simulink model "sampleModel1917"  (R2023a)
settings: Solver=VariableStepAuto  StartTime=0.0  StopTime=10.0  RelTol=1e-3
libraries: hdlsllib x8, simulink x8
settings Model: Creator=user1  LastModifiedBy=user1

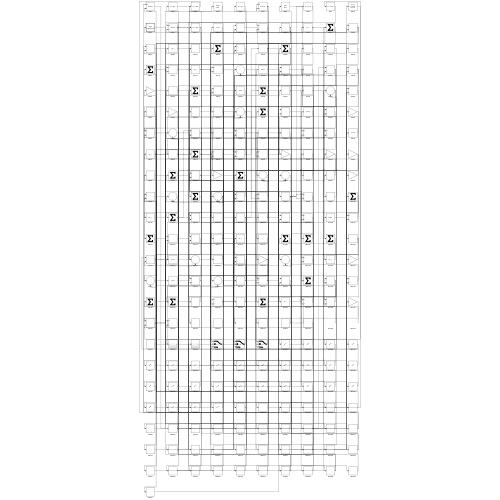
[thumbnail: Simulink's stored preview of the top-level diagram]
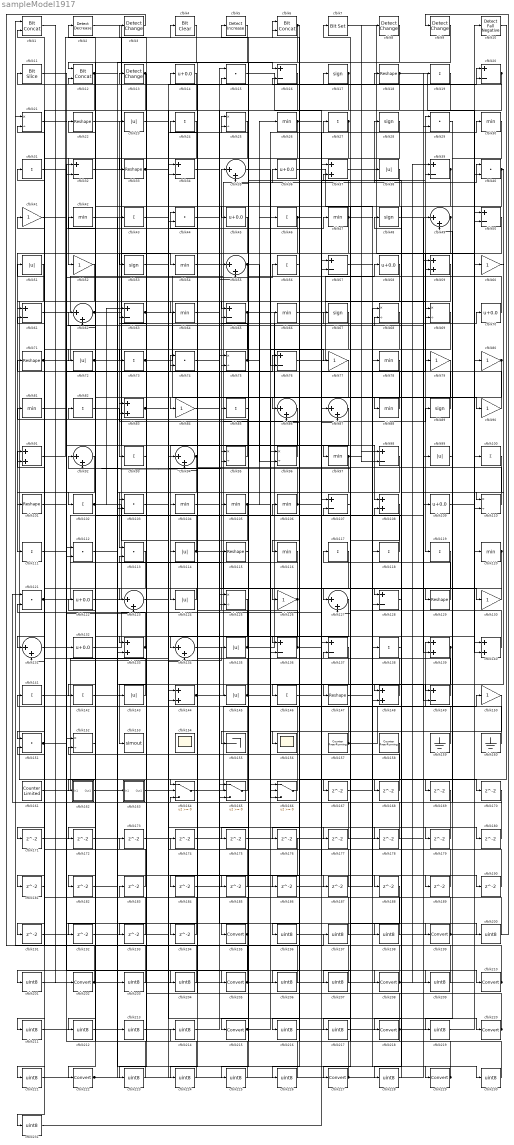
== system sampleModel1917 ==
  cfblk1 : hdlsllib/Logic and Bit Operations/Bit Concat  numInputs=2
  cfblk10 : hdlsllib/Logic and Bit Operations/Detect Fall Negative  vinit=0  OutDataTypeStr=boolean
  cfblk{19,24,27,31,43,46,56,73,82,85,93,100,102,111,117..119,138,141..142,146} (21 alike) : Sum  Inputs=+
  cfblk{18,22,33,71,101,115,129,147} (8 alike) : Reshape
  cfblk{15,29,40,44,74,103,112..113,121,151} (10 alike) : DotProduct  OutDataTypeStr=Inherit: Inherit via internal rule
  cfblk{26,30,42,47,54,64,66,78,81,88,97,104..106,116,120} (16 alike) : MinMax
  cfblk{16,20,32,34,39,50,57,61,63,65,76,98,107,128,136..137,149} (17 alike) : Sum  Inputs=+-
  cfblk{37,59,83,91,108,133,139..140,144,148} (10 alike) : Sum
  cfblk{14,36,45,58,70,109,122,132} (8 alike) : Bias  Bias=0.0  SaturateOnIntegerOverflow=off
  cfblk11 : hdlsllib/Logic and Bit Operations/Bit Slice  lidx=7  ridx=0
  cfblk{21,25,68..69,75,95..96,110,125,152} (10 alike) : Product  Inputs=*/  RndMeth=Zero  SaturateOnIntegerOverflow=on
  cfblk{23,38,51,72,99,114,124,135,143,145} (10 alike) : Abs  SaturateOnIntegerOverflow=off
  cfblk12 : hdlsllib/Logic and Bit Operations/Bit Concat  numInputs=2
  cfblk{35,49,55,62,86..87,92,94,123,127,131,134} (12 alike) : Sum  Inputs=|++
  cfblk{41,52,60,77,79..80,84,90,126,130,150} (11 alike) : Gain
  cfblk{3,8..9,13} (4 alike) : simulink/Logic and Bit Operations/Detect Change  vinit=0  OutDataTypeStr=boolean
      settings: LibrarySourceBlock=|
      | hdlsllib/Logic and Bit
      | Operations/Detect
      | Change
  cfblk153 : ToWorkspace  VariableName=simout  SaveFormat=Timeseries  SampleTime=-1
  cfblk154 : Scope
      settings: Floating=on
  cfblk155 : Terminator
  cfblk156 : Scope
  cfblk157 : hdlsllib/Sources/Counter Free-Running  NumBits=16  tsamp=-1
  cfblk158 : hdlsllib/Sources/Counter Free-Running  NumBits=16  tsamp=-1
  cfblk159 : Ground
  cfblk160 : Ground
  cfblk161 : hdlsllib/Sources/Counter Limited  uplimit=7  tsamp=-1
  cfblk162 : Subsystem
      settings: LibrarySourceBlock=|
      | hdlsllib/Ports &
      | Subsystems/Subsystem
  cfblk163 : Subsystem
      settings: LibrarySourceBlock=|
      | hdlsllib/Ports &
      | Subsystems/Subsystem
  cfblk164 : Switch  SaturateOnIntegerOverflow=off  InputSameDT=off
  cfblk165 : Switch  SaturateOnIntegerOverflow=off  InputSameDT=off
  cfblk166 : Switch  SaturateOnIntegerOverflow=off  InputSameDT=off
  cfblk{167..194} (28 alike) : Delay  SampleTime=1
  cfblk{17,28,48,53,67,89} (6 alike) : Signum
  cfblk{195,199,202,205,208,210,215,218,220,222,227,229} (12 alike) : DataTypeConversion  SaturateOnIntegerOverflow=off  RndMeth=Floor
  cfblk{196..198,200..201,203..204,206..207,209,211..214,216..217,219,221,223..226,228,230..231} (25 alike) : DataTypeConversion  OutDataTypeStr=uint8  SaturateOnIntegerOverflow=off  RndMeth=Floor
  cfblk2 : simulink/Logic and Bit Operations/Detect Decrease  vinit=0.0  OutDataTypeStr=boolean
      settings: LibrarySourceBlock=|
      | hdlsllib/Logic and Bit
      | Operations/Detect
      | Decrease
  cfblk4 : simulink/Logic and Bit Operations/Bit Clear  iBit=0
      settings: LibrarySourceBlock=|
      | hdlsllib/Logic and Bit
      | Operations/Bit Clear
  cfblk5 : simulink/Logic and Bit Operations/Detect Increase  vinit=0.0  OutDataTypeStr=boolean
      settings: LibrarySourceBlock=|
      | hdlsllib/Logic and Bit
      | Operations/Detect
      | Increase
  cfblk6 : hdlsllib/Logic and Bit Operations/Bit Concat  numInputs=2
  cfblk7 : simulink/Logic and Bit Operations/Bit Set  iBit=0
      settings: LibrarySourceBlock=|
      | hdlsllib/Logic and Bit
      | Operations/Bit Set
  wires:
  cfblk75/1 -> cfblk26/1, cfblk65/2
  cfblk24/1 -> cfblk52/1
  cfblk140/1 -> cfblk92/1
  cfblk91/1 -> cfblk4/1
  cfblk51/1 -> cfblk164/1
  cfblk60/1 -> cfblk147/1
  cfblk76/1 -> cfblk58/1
  cfblk7/1 -> cfblk119/1
  cfblk144/1 -> cfblk36/1, cfblk55/2
  cfblk78/1 -> cfblk102/1
  cfblk134/1 -> cfblk89/1
  cfblk135/1 -> cfblk70/1, cfblk74/1
  cfblk146/1 -> cfblk87/1
  cfblk122/1 -> cfblk6/1
  cfblk98/1 -> cfblk113/1
  cfblk31/1 -> cfblk132/1
  cfblk80/1 -> cfblk127/1, cfblk156/1
  cfblk136/1 -> cfblk35/1, cfblk30/1
  cfblk37/1 -> cfblk80/1
  cfblk61/1 -> cfblk28/1
  cfblk89/1 -> cfblk29/1
  cfblk2/1 -> cfblk54/1
  cfblk116/1 -> cfblk113/2
  cfblk39/1 -> cfblk72/1, cfblk185/1
  cfblk45/1 -> cfblk84/1
  cfblk114/1 -> cfblk126/1, cfblk62/2
  cfblk115/1 -> cfblk25/1
  cfblk90/1 -> cfblk44/1
  cfblk139/1 -> cfblk148/2, cfblk206/1
  cfblk73/1 -> cfblk40/1, cfblk90/1
  cfblk161/1 -> cfblk135/1
  cfblk82/1 -> cfblk93/1
  cfblk5/1 -> cfblk162/1(In1)
  cfblk166/1 -> cfblk24/1
  cfblk46/1 -> cfblk111/1, cfblk190/1
  cfblk143/1 -> cfblk71/1
  cfblk109/1 -> cfblk60/1
  cfblk119/1 -> cfblk128/1
  cfblk4/1 -> cfblk12/1
  cfblk13/1 -> cfblk61/1, cfblk73/1
  cfblk165/1 -> cfblk62/1
  cfblk148/1 -> cfblk81/1
  cfblk53/1 -> cfblk20/1
  cfblk43/1 -> cfblk210/1
  cfblk106/1 -> cfblk82/1, cfblk39/2
  cfblk160/1 -> cfblk91/1
  cfblk8/1 -> cfblk136/1
  cfblk18/1 -> cfblk120/1, cfblk86/1
  cfblk105/1 -> cfblk124/1, cfblk46/1, cfblk27/1
  cfblk142/1 -> cfblk153/1
  cfblk88/1 -> cfblk31/1
  cfblk121/1 -> cfblk49/1, cfblk115/1
  cfblk83/1 -> cfblk143/1, cfblk140/2
  cfblk34/1 -> cfblk130/1
  cfblk58/1 -> cfblk65/1
  cfblk32/1 -> cfblk138/1
  cfblk137/1 -> cfblk146/1
  cfblk157/1 -> cfblk106/1, cfblk150/1
  cfblk69/1 -> cfblk134/1
  cfblk147/1 -> cfblk78/1
  cfblk9/1 -> cfblk195/1
  cfblk22/1 -> cfblk166/1
  cfblk21/1 -> cfblk205/1
  cfblk40/1 -> cfblk88/1, cfblk110/1, cfblk148/1
  cfblk104/1 -> cfblk145/1
  cfblk97/1 -> cfblk127/2, cfblk98/1, cfblk98/2, cfblk8/1, cfblk194/1
  cfblk26/1 -> cfblk45/1, cfblk179/1
  cfblk6/1 -> cfblk184/1, cfblk226/1
  cfblk113/1 -> cfblk131/1
  cfblk57/1 -> cfblk229/1
  cfblk164/1 -> cfblk139/1
  cfblk124/1 -> cfblk123/1
  cfblk1/1 -> cfblk202/1
  cfblk52/1 -> cfblk101/1
  cfblk133/1 -> cfblk121/2, cfblk193/1
  cfblk96/1 -> cfblk23/1
  cfblk44/1 -> cfblk75/1
  cfblk16/1 -> cfblk33/1
  cfblk49/1 -> cfblk144/2, cfblk94/2
  cfblk63/1 -> cfblk139/2, cfblk103/1
  cfblk159/1 -> cfblk117/1
  cfblk77/1 -> cfblk166/2
  cfblk111/1 -> cfblk47/1
  cfblk129/1 -> cfblk17/1
  cfblk100/1 -> cfblk218/1
  cfblk15/1 -> cfblk107/1
  cfblk66/1 -> cfblk69/1
  cfblk131/1 -> cfblk56/1
  cfblk27/1 -> cfblk53/1, cfblk191/1
  cfblk132/1 -> cfblk79/1
  cfblk87/1 -> cfblk114/1
  cfblk23/1 -> cfblk18/1
  cfblk65/1 -> cfblk140/1, cfblk181/1
  cfblk42/1 -> cfblk208/1
  cfblk41/1 -> cfblk97/1
  cfblk14/1 -> cfblk34/2
  cfblk130/1 -> cfblk129/1
  cfblk102/1 -> cfblk134/2, cfblk63/1
  cfblk112/1 -> cfblk199/1
  cfblk95/1 -> cfblk13/1
  cfblk117/1 -> cfblk131/2
  cfblk152/1 -> cfblk222/1
  cfblk141/1 -> cfblk20/2
  cfblk11/1 -> cfblk123/2
  cfblk55/1 -> cfblk96/2, cfblk172/1
  cfblk138/1 -> cfblk48/1
  cfblk163/1(Out1) -> cfblk220/1
  cfblk110/1 -> cfblk75/2
  cfblk86/1 -> cfblk104/1
  cfblk67/1 -> cfblk116/1
  cfblk99/1 -> cfblk59/2
  cfblk48/1 -> cfblk99/1
  cfblk103/1 -> cfblk95/1
  cfblk33/1 -> cfblk177/1, cfblk178/1
  cfblk62/1 -> cfblk108/1, cfblk192/1
  cfblk54/1 -> cfblk165/1
  cfblk30/1 -> cfblk149/1
  cfblk50/1 -> cfblk215/1
  cfblk123/1 -> cfblk25/2
  cfblk151/1 -> cfblk68/2, cfblk76/1
  cfblk118/1 -> cfblk83/1
  cfblk12/1 -> cfblk151/1, cfblk16/1, cfblk149/2
  cfblk150/1 -> cfblk166/3
  cfblk71/1 -> cfblk29/2, cfblk170/1
  cfblk35/1 -> cfblk77/1
  cfblk72/1 -> cfblk67/1, cfblk187/1
  cfblk17/1 -> cfblk32/2, cfblk165/3
  cfblk94/1 -> cfblk92/2, cfblk103/2
  cfblk79/1 -> cfblk142/1
  cfblk38/1 -> cfblk227/1
  cfblk120/1 -> cfblk175/1, cfblk219/1
  cfblk47/1 -> cfblk11/1, cfblk76/2, cfblk189/1
  cfblk20/1 -> cfblk86/2, cfblk16/2, cfblk176/1
  cfblk25/1 -> cfblk64/1
  cfblk36/1 -> cfblk118/1
  cfblk145/1 -> cfblk69/2, cfblk83/2
  cfblk70/1 -> cfblk5/1
  cfblk149/1 -> cfblk105/1
  cfblk59/1 -> cfblk133/1
  cfblk126/1 -> cfblk164/2, cfblk155/1, cfblk63/2
  cfblk107/1 -> cfblk167/1
  cfblk167/1 -> cfblk68/1
  cfblk10/1 -> cfblk168/1
  cfblk168/1 -> cfblk12/2
  cfblk29/1 -> cfblk169/1
  cfblk169/1 -> cfblk121/1
  cfblk170/1 -> cfblk164/3
  cfblk92/1 -> cfblk171/1
  cfblk171/1 -> cfblk144/1
  cfblk173/1 -> cfblk59/1
  cfblk174/1 -> cfblk87/2
  cfblk175/1 -> cfblk96/1
  cfblk177/1 -> cfblk95/2
  cfblk178/1 -> cfblk137/1
  cfblk179/1 -> cfblk32/1
  cfblk84/1 -> cfblk180/1
  cfblk180/1 -> cfblk49/2
  cfblk127/1 -> cfblk182/1
  cfblk183/1 -> cfblk61/2
  cfblk184/1 -> cfblk128/2
  cfblk185/1 -> cfblk34/1
  cfblk56/1 -> cfblk186/1
  cfblk187/1 -> cfblk35/2
  cfblk64/1 -> cfblk188/1
  cfblk189/1 -> cfblk165/2
  cfblk190/1 -> cfblk108/2
  cfblk191/1 -> cfblk94/1
  cfblk192/1 -> cfblk133/2
  cfblk193/1 -> cfblk151/2
  cfblk194/1 -> cfblk41/1
  cfblk195/1 -> cfblk51/1, cfblk211/1
  cfblk158/1 -> cfblk196/1
  cfblk196/1 -> cfblk9/1
  cfblk3/1 -> cfblk197/1
  cfblk197/1 -> cfblk14/1
  cfblk74/1 -> cfblk198/1
  cfblk198/1 -> cfblk3/1
  cfblk199/1 -> cfblk40/2, cfblk141/1
  cfblk101/1 -> cfblk200/1
  cfblk200/1 -> cfblk112/1
  cfblk181/1 -> cfblk201/1
  cfblk201/1 -> cfblk112/2
  cfblk202/1 -> cfblk66/1, cfblk55/1, cfblk109/1, cfblk91/2
  cfblk172/1 -> cfblk203/1
  cfblk203/1 -> cfblk1/1
  cfblk176/1 -> cfblk204/1
  cfblk204/1 -> cfblk1/2
  cfblk205/1 -> cfblk74/2, cfblk10/1
  cfblk206/1 -> cfblk21/1
  cfblk188/1 -> cfblk207/1
  cfblk207/1 -> cfblk21/2
  cfblk208/1 -> cfblk110/2, cfblk39/1, cfblk7/1
  cfblk81/1 -> cfblk209/1
  cfblk209/1 -> cfblk42/1
  cfblk210/1 -> cfblk122/1, cfblk22/1
  cfblk211/1 -> cfblk43/1
  cfblk125/1 -> cfblk212/1
  cfblk212/1 -> cfblk15/1
  cfblk162/1(Out1) -> cfblk213/1
  cfblk213/1 -> cfblk125/1
  cfblk214/1 -> cfblk125/2
  cfblk215/1 -> cfblk136/2, cfblk15/2
  cfblk186/1 -> cfblk216/1
  cfblk216/1 -> cfblk50/1
  cfblk108/1 -> cfblk217/1
  cfblk217/1 -> cfblk50/2
  cfblk218/1 -> cfblk214/1, cfblk174/1, cfblk173/1
  cfblk219/1 -> cfblk100/1
  cfblk220/1 -> cfblk137/2, cfblk107/2
  cfblk68/1 -> cfblk221/1
  cfblk221/1 -> cfblk163/1(In1)
  cfblk222/1 -> cfblk44/2, cfblk19/1
  cfblk93/1 -> cfblk223/1
  cfblk223/1 -> cfblk152/1
  cfblk28/1 -> cfblk224/1
  cfblk224/1 -> cfblk152/2
  cfblk85/1 -> cfblk225/1
  cfblk225/1 -> cfblk183/1
  cfblk226/1 -> cfblk85/1
  cfblk227/1 -> cfblk6/2, cfblk37/1
  cfblk128/1 -> cfblk228/1
  cfblk228/1 -> cfblk38/1
  cfblk229/1 -> cfblk37/2, cfblk2/1
  cfblk182/1 -> cfblk230/1
  cfblk230/1 -> cfblk57/1
  cfblk19/1 -> cfblk231/1
  cfblk231/1 -> cfblk57/2

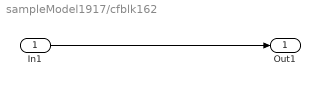
== system sampleModel1917/cfblk162 ==
  In1 : Inport
  Out1 : Outport
  wires:
  In1/1 -> Out1/1

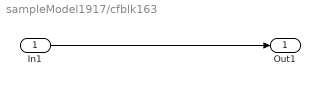
== system sampleModel1917/cfblk163 ==
  In1 : Inport
  Out1 : Outport
  wires:
  In1/1 -> Out1/1
